simulink model "VFD"  (R2024b)
settings: Solver=VariableStepAuto  StartTime=0.0  StopTime=10/50  RelTol=1e-3
values from neighbouring files (symbols this model uses):
  C = (1-d)/(8*L*(2/31)*freq*freq)    (= 6.25e-05)    [variables.m]
  fnew = 33    [variables.m]
  freq = 50    [variables.m]
  r = 1000    [variables.m]
undefined symbols (not defined in the file or in its folder): Down, Up
libraries: fl_lib x38, nesl_utility x27, ee_lib x12, eePwmGenerator x3, simulink x1
settings Model: Creator=nilab  LastModifiedBy=nilab
settings DebuggingCC: ReadBeforeWriteMsg=DisableAll  WriteAfterWriteMsg=DisableAll  WriteAfterReadMsg=DisableAll  MultiTaskDSMMsg=none
settings ModelReferenceCC: UpdateModelReferenceTargets=IfOutOfDate
settings SFSimCC: SFSimEcho=off

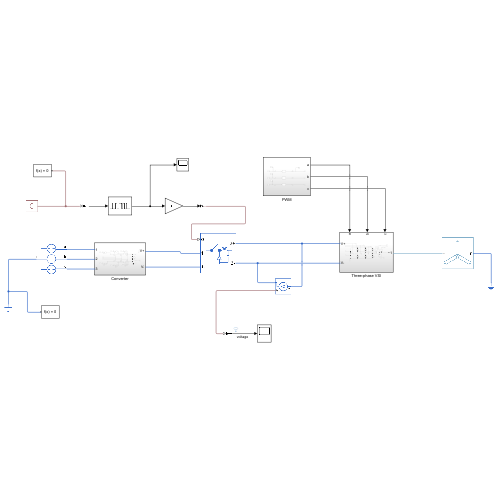
[thumbnail: Simulink's stored preview of the top-level diagram]
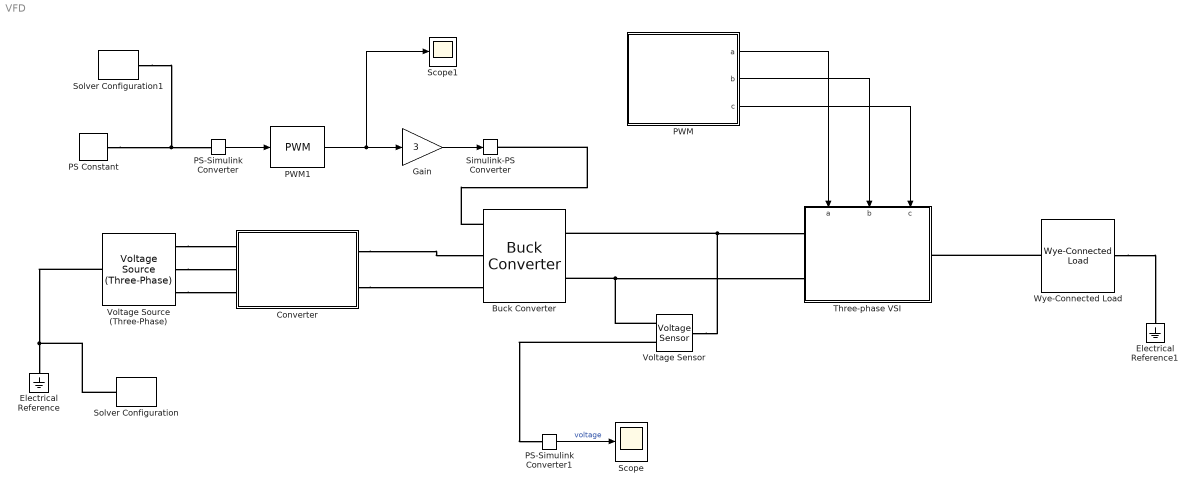
== system VFD ==
  Buck Converter : ee_lib/Semiconductors & Converters/Converters/Buck Converter  port_option=ee.enum.controlport.ps  device_type=ee.enum.converters.switchingdevice.ideal  Vf=0.8 V  Ron=0.001 Ohm  Rds=0.001 Ohm  Goff=1e-5 1/Ohm  Vgt=1 V  Vgt_off=-1 V  Ih=1 A  Vth=2 V  K=0  diode_param=ee.enum.converters.protectiondiode.nodynamics  diode_Vf=0.8 V  diode_Ron=0.001 Ohm  diode_Goff=1e-5 1/Ohm  diode_C=50 nF  diode_iRM=-235 A  diode_iF=300 A  diode_idot=-50 A/us  diode_trr_param=ee.enum.converters.diodetrr.trr_factor  diode_trr_factor=3  diode_trr=15 us  diode_Qrr=1500 s*uA  Lf=L H  Rl=0 Ohm  Cf=C*1e6 uF  Rf=1e-6 Ohm  snubber_type=ee.enum.converters.snubber.exclude  Cs=1e-7 F  Rs=0.1 Ohm  iL_specify=off  iL_priority=High  iL=0 A  iL_nominal_specify=off  iL_nominal_value=1  iL_nominal_unit=A  vc_specify=off  vc_priority=High  vc=0 V  vc_nominal_specify=off  vc_nominal_value=1  vc_nominal_unit=V
      settings: InternalSimscapePortConfiguration="{\"Bottom\":[],\"Left\":[{\"id\":\"G\",\"label\":\"G\",\"type\":\"input\"},{\"id\":\"p1\",\"label\":\"1+\",\"type\":\"foundation.electrical.electrical\"},{\"id\":\"n1\",\"label\":\"1-\",\"type\":\"foundation.electrical.electrical\"}],\"Right\":[{\"id\":\"p2\",\"label\":\"2+\",\"type\":\"foundation.electrical.electrical\"},{\"id\":\"n2\",\"label\":\"2-\",\"type\":\"foundation.electrical.electrical\"}],\"Top\":[]}"
  Converter : Subsystem
  Electrical Reference : fl_lib/Electrical/Electrical Elements/Electrical Reference
  Electrical Reference1 : fl_lib/Electrical/Electrical Elements/Electrical Reference
  Gain : Gain  Gain=3
  PS Constant : fl_lib/Physical Signals/Sources/PS Constant  constant=d
  PS-Simulink Converter : nesl_utility/PS-Simulink Converter  PhysicalDomain=network_engine_domain  SubClassName=ps_output  LeftPortType=input  RightPortType=output  PseudoPeriodic=off  Frequencies=[]  VectorFormat=inherit  Unit=inherit  AffineConversion=off
  PS-Simulink Converter1 : nesl_utility/PS-Simulink Converter  PhysicalDomain=network_engine_domain  SubClassName=ps_output  LeftPortType=input  RightPortType=output  PseudoPeriodic=off  Frequencies=[]  VectorFormat=inherit  Unit=inherit  AffineConversion=off
  PWM : Subsystem
  PWM1 : simulink/Discontinuities/PWM  DisableCoverage=on  Period=1/fnew  InitialDelay=0  DisallowZeroDutyCycle=off  RunAtFixedTimeIntervals=off  SampleTime=0.1
  Scope : Scope
  Scope1 : Scope
  Simulink-PS Converter : nesl_utility/Simulink-PS Converter  PhysicalDomain=network_engine_domain  SubClassName=ps_input  LeftPortType=input  RightPortType=output  PseudoPeriodic=off  Frequencies=[]  NoiseDistribution=none  NoiseParameters=[]  Unit=1  AffineConversion=off  FilteringAndDerivatives=provide  SimscapeFilterOrder=1  InputFilterTimeConstant=0.001  UdotUserProvided=0
  Solver Configuration : nesl_utility/Solver Configuration  PhysicalDomain=network_engine_domain  SubClassName=solver  LeftPortType=input  RightPortType=generic  Tones=[]  Harmonics=[]  SimulateNoise=off  Profile=off  UseLocalSampling=off  EnableSwitchedLinearOptims=on  FrequencyDomain=off  UseCCode=off  RelTol=0.001  AbsTol=0.001  MinStep=1e-09  ToWorkspace=off  RevertToSquareIcSolve=off  NumHomotopyIterations=100  PhasorMode=off  PhasorModeNumHarmonics=1  ConsistencySolver=NEWTON_XTOL_AFTER_FTOL  IndexReductionMethod=DerivativeReplacement  DoDC=off  ResidualTolerance=1e-09  ConsistencyTolSource=GLOBAL  ConsistencyAbsTol=0.001  ConsistencyRelTol=0.001  ConsistencyTolFactor=0.001  UseLocalSolver=off  LocalSolverChoice=NE_BACKWARD_EULER_ADVANCER  ResolveIndetEquations=on  FunctionEvalNumThread=1  LocalSolverSampleTime=0.001  DoFixedCost=off  MaxNonlinIter=3  MaxModeIter=2  ComputeImpulses=off  ImpulseIterations=2  LinearAlgebra=auto  LinearAlgebraNumThread=0  EquationFormulation=NE_TIME_EF  DelaysMemoryBudget=1024  AutomaticFiltering=on  FilteringTimeConstant=0.001  PartitionStorageMethod=AS_NEEDED  PartitionMemoryBudget=1024  PartitionMethod=ROBUST  MultibodyUseLocalSolver=off  MultibodyLocalSolverChoice=ODE1  MultibodyLocalSolverSampleTime=0.001
  Solver Configuration1 : nesl_utility/Solver Configuration  PhysicalDomain=network_engine_domain  SubClassName=solver  LeftPortType=input  RightPortType=generic  Tones=[]  Harmonics=[]  SimulateNoise=off  Profile=off  UseLocalSampling=off  EnableSwitchedLinearOptims=on  FrequencyDomain=off  UseCCode=off  RelTol=0.001  AbsTol=0.001  MinStep=1e-09  ToWorkspace=off  RevertToSquareIcSolve=off  NumHomotopyIterations=100  PhasorMode=off  PhasorModeNumHarmonics=1  ConsistencySolver=NEWTON_XTOL_AFTER_FTOL  IndexReductionMethod=DerivativeReplacement  DoDC=off  ResidualTolerance=1e-09  ConsistencyTolSource=GLOBAL  ConsistencyAbsTol=0.001  ConsistencyRelTol=0.001  ConsistencyTolFactor=0.001  UseLocalSolver=off  LocalSolverChoice=NE_BACKWARD_EULER_ADVANCER  ResolveIndetEquations=on  FunctionEvalNumThread=1  LocalSolverSampleTime=0.001  DoFixedCost=off  MaxNonlinIter=3  MaxModeIter=2  ComputeImpulses=off  ImpulseIterations=2  LinearAlgebra=auto  LinearAlgebraNumThread=0  EquationFormulation=NE_TIME_EF  DelaysMemoryBudget=1024  AutomaticFiltering=on  FilteringTimeConstant=0.001  PartitionStorageMethod=AS_NEEDED  PartitionMemoryBudget=1024  PartitionMethod=ROBUST  MultibodyUseLocalSolver=off  MultibodyLocalSolverChoice=ODE1  MultibodyLocalSolverSampleTime=0.001
  Three-phase VSI : Subsystem
      settings: PortSchema="{\"entries\":[{\"content\":{\"sides\":[{\"content\":{\"connectorIds\":[\"LConn1\",\"LConn2\"]},\"type\":\"ConnectorPlacement.EquallySpacedRectSide\",\"uuid\":\"2b5e637c-93e3-4064-8bf6-4f52f0e07da4\"},{\"content\":{\"connectorIds\":[\"RConn1\"],\"side\":\"RIGHT\"},\"type\":\"ConnectorPlacement.EquallySpacedRectSide\",\"uuid\":\"63a19c73-cdb8-4eaa-8504-93f2b55e949d\"},{\"content\":{\"connectorIds\":[\"In1\",\"In2\",\"In3\"],\"side\":\"TOP\"},\"type\":\"ConnectorPlacement.EquallySpacedRectSide\",\"uuid\":\"d4653da6-a00c-414a-9a01-4f896c6dc2e2\"}]},\"type\":\"ConnectorPlacement.EquallySpacedConnector\",\"uuid\":\"c4601345-6e28-4ab4-9b60-968efd743150\"}],\"packageUris\":[\"http://schema.mathworks.com/mf0/Connector/R2020b\"],\"version\":\"1.0\"}"
  Voltage Source (Three-Phase) : ee_lib/Sources/Voltage Source (Three-Phase)  vline_rms=220/sqrt(3) V  shift=0 deg  freq=50 Hz  impedance_option=1  SShortCircuit=1e6 A*V  XR=15  R=0.01 Ohm  L=3.97e-4 H  harmonic_option=0  harmonic_orders=[5, 7, 11, 13]  harmonic_ratios=[.1, .1, .1, .1]  G_parasitic=0 1/Ohm  I_specify=off  I_priority=None  I=[0, 0, 0] A  I_nominal_specify=off  I_nominal_value=1  I_nominal_unit=A
      settings: InternalSimscapePortConfiguration="{\"Bottom\":[],\"Left\":[{\"id\":\"n\",\"label\":\"n\",\"type\":\"foundation.electrical.electrical\"}],\"Right\":[{\"id\":\"a\",\"label\":\"a\",\"type\":\"foundation.electrical.electrical\"},{\"id\":\"b\",\"label\":\"b\",\"type\":\"foundation.electrical.electrical\"},{\"id\":\"c\",\"label\":\"c\",\"type\":\"foundation.electrical.electrical\"}],\"Top\":[]}"
  Voltage Sensor : fl_lib/Electrical/Electrical Sensors/Voltage Sensor
  Wye-Connected Load : ee_lib/Passive/RLC Assemblies/Wye-Connected Load  port_option=ee.enum.threePhasePort.composite  parameterization=ee.enum.rlc.parameterization.direct  component_structure=ee.enum.rlc.structure.R  component_structure_PQ=ee.enum.rlc.structure.R  R=r Ohm  L=1e-3 H  C=1e-6 F  VRated=24e3 V  FRated=60 Hz  P=1e3 W  Qpos=1e2 A*V  Qneg=-1e2 A*V  R_parasitic=1e-6 Ohm  G_parasitic=1e-6 1/Ohm  R_parasitic_PQ=1e-6 Ohm  G_parasitic_PQ=1e-6 1/Ohm  Vmag0=24e3 V  Vang0=0 deg  Freq0=60 Hz  IL_specify=off  IL_priority=High  IL=[0, 0, 0] A  IL_nominal_specify=off  IL_nominal_value=1  IL_nominal_unit=A  VC_specify=off  VC_priority=High  VC=[0, 0, 0] V  VC_nominal_specify=off  VC_nominal_value=1  VC_nominal_unit=V
  wires:
  PS-Simulink Converter/1 -> PWM1/1
  PWM/1(a) -> Three-phase VSI/1(a)
  PWM/2(b) -> Three-phase VSI/2(b)
  PWM/3(c) -> Three-phase VSI/3(c)
  PS-Simulink Converter1/1 -> Scope/1  "voltage"
  PWM1/1 -> Gain/1, Scope1/1
  Gain/1 -> Simulink-PS Converter/1
  connections:
  Voltage Source (Three-Phase)/RConn2 -- Converter/LConn2
  Voltage Source (Three-Phase)/RConn1 -- Converter/LConn1
  Voltage Source (Three-Phase)/RConn3 -- Converter/LConn3
  Voltage Source (Three-Phase)/LConn1 -- Solver Configuration/RConn1 -- Electrical Reference/LConn1
  Buck Converter/LConn1 -- Simulink-PS Converter/RConn1
  PS Constant/RConn1 -- PS-Simulink Converter/LConn1 -- Solver Configuration1/RConn1
  Voltage Sensor/RConn2 -- Three-phase VSI/LConn2 -- Buck Converter/RConn2
  Voltage Sensor/RConn1 -- PS-Simulink Converter1/LConn1
  Voltage Sensor/LConn1 -- Three-phase VSI/LConn1 -- Buck Converter/RConn1
  Converter/RConn2 -- Buck Converter/LConn3
  Converter/RConn1 -- Buck Converter/LConn2
  Wye-Connected Load/LConn1 -- Three-phase VSI/RConn1
  Wye-Connected Load/RConn1 -- Electrical Reference1/LConn1

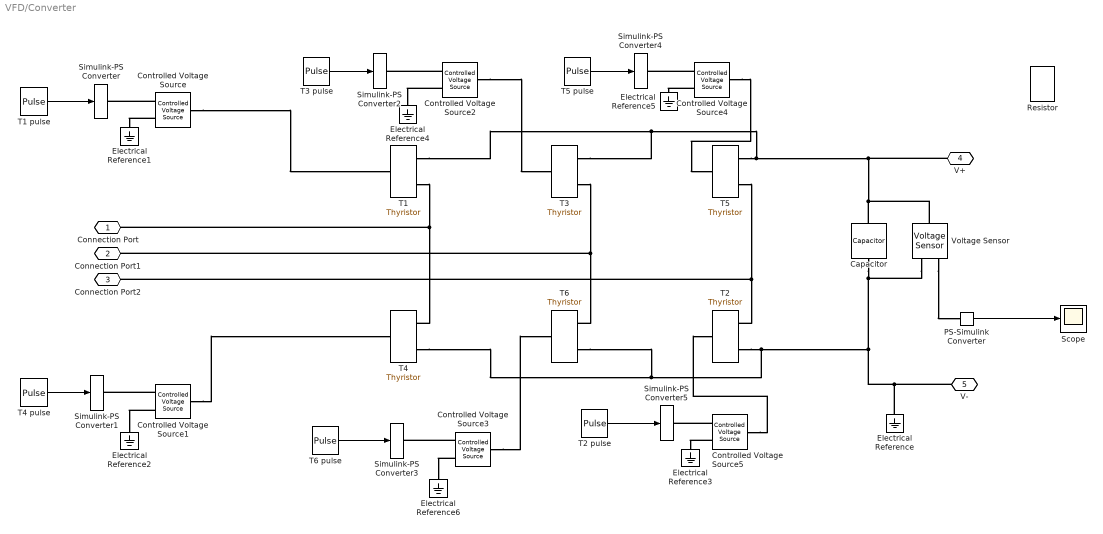
== system VFD/Converter ==
  Capacitor : fl_lib/Electrical/Electrical Elements/Capacitor  c=100 uF  r=1e-6 Ohm  g=0 1/Ohm  i_specify=off  i_priority=None  i=0 A  i_nominal_specify=off  i_nominal_value=1  i_nominal_unit=A  v_specify=off  v_priority=None  v=0 V  v_nominal_specify=off  v_nominal_value=1  v_nominal_unit=V  vc_specify=off  vc_priority=High  vc=0 V  vc_nominal_specify=off  vc_nominal_value=1  vc_nominal_unit=V
  Controlled Voltage Source{,1..5} (6 alike) : fl_lib/Electrical/Electrical Sources/Controlled Voltage Source
  Electrical Reference{,1..6} (7 alike) : fl_lib/Electrical/Electrical Elements/Electrical Reference
  PS-Simulink Converter : nesl_utility/PS-Simulink Converter  PhysicalDomain=network_engine_domain  SubClassName=ps_output  LeftPortType=input  RightPortType=output  PseudoPeriodic=off  Frequencies=[]  VectorFormat=inherit  Unit=inherit  AffineConversion=off
  Resistor : fl_lib/Electrical/Electrical Elements/Resistor  R=1 Ohm  i_specify=off  i_priority=None  i=0 A  i_nominal_specify=off  i_nominal_value=1  i_nominal_unit=A  v_specify=off  v_priority=None  v=0 V  v_nominal_specify=off  v_nominal_value=1  v_nominal_unit=V
  Scope : Scope
  Simulink-PS Converter{,1..5} (6 alike) : nesl_utility/Simulink-PS Converter  PhysicalDomain=network_engine_domain  SubClassName=ps_input  LeftPortType=input  RightPortType=output  PseudoPeriodic=off  Frequencies=[]  NoiseDistribution=none  NoiseParameters=[]  Unit=1  AffineConversion=off  FilteringAndDerivatives=zero  SimscapeFilterOrder=1  InputFilterTimeConstant=0.001  UdotUserProvided=1
  T{1..6} (6 alike) : ee_lib/Semiconductors & Converters/Thyristor  model_type=ee.enum.semiconductors.thyristorModelType.equations  v_on=1.2 V  i_on=1 A  VT_vec=[.75, 1, 1.25, 1.5, 1.75, 2, 2.25] V  IT_vec=[.015, .22, .75, 1.4, 2, 2.75, 3.45] A  IDRM=0.01 mA  VDRM=400 V  i_H=1 mA  Tmeas=25 degC  i_GT=3 uA  v_GT=0.6 V  V_D=12 V  R=120 Ohm  dVdt=150 V/us  R_GK=1000 Ohm  TF_NPN_parameterization=1  T_d=2 us  i_d=10 mA  TF_NPN=0.3 us  TF_PNP_parameterization=1  TF_PNP=0.3 us  t_on_delay=0 s  t_on_curr=1 mA  t_on_rise=0 s  Rs=87 kOhm  Rgate=10 Ohm  Gain=10  ig_specify=off  ig_priority=None  ig=0 A  ig_nominal_specify=off  ig_nominal_value=1  ig_nominal_unit=A  ia_specify=off  ia_priority=None  ia=0 A  ia_nominal_specify=off  ia_nominal_value=1  ia_nominal_unit=A  vgk_specify=off  vgk_priority=None  vgk=0 V  vgk_nominal_specify=off  vgk_nominal_value=1  vgk_nominal_unit=V  vak_specify=off  vak_priority=None  vak=0 V  vak_nominal_specify=off  vak_nominal_value=1  vak_nominal_unit=V  Q_npn_bc_specify=off  Q_npn_bc_priority=High  Q_npn_bc=0 C  Q_npn_bc_nominal_specify=off  Q_npn_bc_nominal_value=1  Q_npn_bc_nominal_unit=uC  Q_npn_be_specify=off  Q_npn_be_priority=High  Q_npn_be=0 C  Q_npn_be_nominal_specify=off  Q_npn_be_nominal_value=1  Q_npn_be_nominal_unit=uC  Q_pnp_be_specify=off  Q_pnp_be_priority=High  Q_pnp_be=0 C  Q_pnp_be_nominal_specify=off  Q_pnp_be_nominal_value=1  Q_pnp_be_nominal_unit=uC  thermal_network_parameterization=ee.enum.thermalNetworkTopology.junctionCase  Rth=[0, 10] K/W  Rth_Cauer=[1, 3, 10] K/W  Rth_Foster=[4, 6] K/W  thermal_mass_parameterization=ee.enum.thermalNetwork.timeconstant  thermal_mass=[0, 1] J/K  thermal_mass_Cauer=[.1, .3, 1] J/K  thermal_mass_Foster=[1.5, 3] J/K  thermal_time_constant=[0, 10] s  thermal_time_constant_Cauer=[1, 3, 10] s  thermal_time_constant_Foster=[6, 18] s  thermal_mass_initial_temperatures=[25, 25] degC  thermal_mass_initial_temperatures_Cauer=[25, 25, 25] degC  Tvec_initial_Foster=[25, 25, 25, 25] degC
      settings: InternalSimscapePortConfiguration="{\"Bottom\":[],\"Left\":[{\"id\":\"G\",\"label\":\"\",\"type\":\"foundation.electrical.electrical\"}],\"Right\":[{\"id\":\"A\",\"label\":\"\",\"type\":\"foundation.electrical.electrical\"},{\"id\":\"K\",\"label\":\"\",\"type\":\"foundation.electrical.electrical\"}],\"Top\":[]}"
  T1 pulse : DiscretePulseGenerator  PulseType=Time based  Amplitude=2  Period=1/freq  PulseWidth=5  PhaseDelay=1/(12*freq)
  T2 pulse : DiscretePulseGenerator  PulseType=Time based  Amplitude=2  Period=1/freq  PulseWidth=5  PhaseDelay=1/(4*freq)
  T3 pulse : DiscretePulseGenerator  PulseType=Time based  Amplitude=2  Period=1/freq  PulseWidth=5  PhaseDelay=5/(12*freq)
  T4 pulse : DiscretePulseGenerator  PulseType=Time based  Amplitude=2  Period=1/freq  PulseWidth=5  PhaseDelay=7/(12*freq)
  T5 pulse : DiscretePulseGenerator  PulseType=Time based  Amplitude=2  Period=1/freq  PulseWidth=5  PhaseDelay=3/(4*freq)
  T6 pulse : DiscretePulseGenerator  PulseType=Time based  Amplitude=2  Period=1/freq  PulseWidth=5  PhaseDelay=11/(12*freq)
  Voltage Sensor : fl_lib/Electrical/Electrical Sensors/Voltage Sensor
  Connection Port : PMIOPort  Side=Left
  Connection Port1 : PMIOPort  Port=2  Side=Left
  Connection Port2 : PMIOPort  Port=3  Side=Left
  V+ : PMIOPort  Port=4  Side=Right
  V- : PMIOPort  Port=5  Side=Right
  wires:
  T1 pulse/1 -> Simulink-PS Converter/1
  T6 pulse/1 -> Simulink-PS Converter3/1
  T5 pulse/1 -> Simulink-PS Converter4/1
  T2 pulse/1 -> Simulink-PS Converter5/1
  T3 pulse/1 -> Simulink-PS Converter2/1
  PS-Simulink Converter/1 -> Scope/1
  T4 pulse/1 -> Simulink-PS Converter1/1
  connections:
  T5/RConn1 -- Connection Port2/RConn1 -- T2/RConn2
  T6/RConn2 -- Connection Port1/RConn1 -- T3/RConn1
  T1/RConn1 -- T4/RConn2 -- Connection Port/RConn1
  Controlled Voltage Source5/LConn1 -- T2/LConn1
  Controlled Voltage Source3/RConn2 -- Electrical Reference6/LConn1
  Voltage Sensor/RConn1 -- PS-Simulink Converter/LConn1
  Controlled Voltage Source1/RConn1 -- Simulink-PS Converter1/RConn1
  Controlled Voltage Source5/RConn1 -- Simulink-PS Converter5/RConn1
  Controlled Voltage Source4/RConn2 -- Electrical Reference5/LConn1
  Controlled Voltage Source3/RConn1 -- Simulink-PS Converter3/RConn1
  Controlled Voltage Source4/LConn1 -- T5/LConn1
  Controlled Voltage Source3/LConn1 -- T6/LConn1
  Controlled Voltage Source1/LConn1 -- T4/LConn1
  Controlled Voltage Source5/RConn2 -- Electrical Reference3/LConn1
  Controlled Voltage Source2/RConn1 -- Simulink-PS Converter2/RConn1
  Controlled Voltage Source/RConn2 -- Electrical Reference1/LConn1
  Controlled Voltage Source1/RConn2 -- Electrical Reference2/LConn1
  Controlled Voltage Source2/LConn1 -- T3/LConn1
  Controlled Voltage Source4/RConn1 -- Simulink-PS Converter4/RConn1
  Controlled Voltage Source2/RConn2 -- Electrical Reference4/LConn1
  Controlled Voltage Source/RConn1 -- Simulink-PS Converter/RConn1
  Controlled Voltage Source/LConn1 -- T1/LConn1
  T6/RConn1 -- T4/RConn1 -- Electrical Reference/LConn1 -- V-/RConn1 -- Capacitor/RConn1 -- Voltage Sensor/RConn2 -- T2/RConn1
  T3/RConn2 -- T1/RConn2 -- V+/RConn1 -- Capacitor/LConn1 -- Voltage Sensor/LConn1 -- T5/RConn2

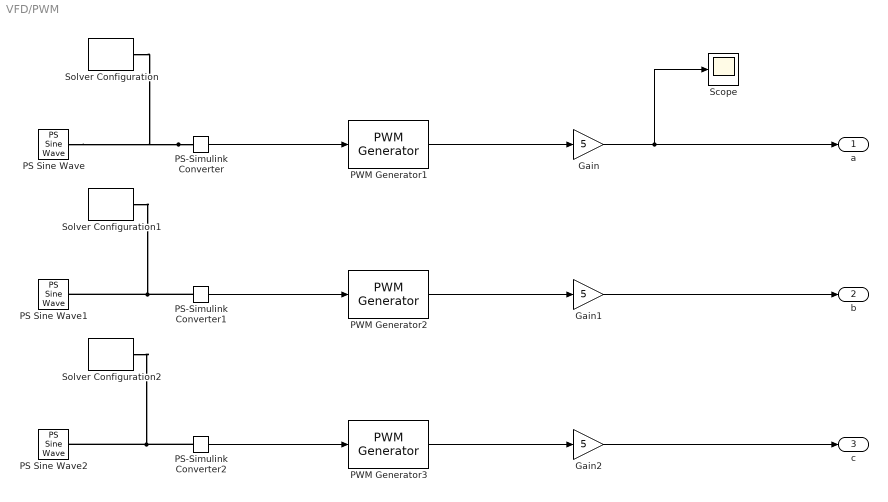
== system VFD/PWM ==
  Gain : Gain  Gain=5
  Gain1 : Gain  Gain=5
  Gain2 : Gain  Gain=5
  PS Sine Wave : fl_lib/Physical Signals/Sources/PS Sine Wave  amplitude=1  bias=0  frequency_spec=foundation.enum.frequencySpec.frequencySI  frequency_SI=fnew Hz  frequency_angular=1 rad/s  phase=0 rad
      settings: InternalSimscapePortConfiguration="{\"Bottom\":[],\"Left\":[],\"Right\":[{\"id\":\"O\",\"label\":\"\",\"type\":\"output\"}],\"Top\":[]}"
  PS Sine Wave1 : fl_lib/Physical Signals/Sources/PS Sine Wave  amplitude=1  bias=0  frequency_spec=foundation.enum.frequencySpec.frequencySI  frequency_SI=fnew Hz  frequency_angular=1 rad/s  phase=-120 deg
      settings: InternalSimscapePortConfiguration="{\"Bottom\":[],\"Left\":[],\"Right\":[{\"id\":\"O\",\"label\":\"\",\"type\":\"output\"}],\"Top\":[]}"
  PS Sine Wave2 : fl_lib/Physical Signals/Sources/PS Sine Wave  amplitude=1  bias=0  frequency_spec=foundation.enum.frequencySpec.frequencySI  frequency_SI=fnew Hz  frequency_angular=1 rad/s  phase=120 deg
      settings: InternalSimscapePortConfiguration="{\"Bottom\":[],\"Left\":[],\"Right\":[{\"id\":\"O\",\"label\":\"\",\"type\":\"output\"}],\"Top\":[]}"
  PS-Simulink Converter : nesl_utility/PS-Simulink Converter  PhysicalDomain=network_engine_domain  SubClassName=ps_output  LeftPortType=input  RightPortType=output  PseudoPeriodic=off  Frequencies=[]  VectorFormat=inherit  Unit=inherit  AffineConversion=off
  PS-Simulink Converter1 : nesl_utility/PS-Simulink Converter  PhysicalDomain=network_engine_domain  SubClassName=ps_output  LeftPortType=input  RightPortType=output  PseudoPeriodic=off  Frequencies=[]  VectorFormat=inherit  Unit=inherit  AffineConversion=off
  PS-Simulink Converter2 : nesl_utility/PS-Simulink Converter  PhysicalDomain=network_engine_domain  SubClassName=ps_output  LeftPortType=input  RightPortType=output  PseudoPeriodic=off  Frequencies=[]  VectorFormat=inherit  Unit=inherit  AffineConversion=off
  PWM Generator1 : eePwmGenerator/PWM Generator  CarrCount=Up-Down  Tper=0.0005  Tdelay=0  Ts=0
  PWM Generator2 : eePwmGenerator/PWM Generator  CarrCount=Up-Down  Tper=0.0005  Tdelay=0  Ts=0
  PWM Generator3 : eePwmGenerator/PWM Generator  CarrCount=Up-Down  Tper=0.0005  Tdelay=0  Ts=0
  Scope : Scope
  Solver Configuration : nesl_utility/Solver Configuration  PhysicalDomain=network_engine_domain  SubClassName=solver  LeftPortType=input  RightPortType=generic  Tones=[]  Harmonics=[]  SimulateNoise=off  Profile=off  UseLocalSampling=off  EnableSwitchedLinearOptims=on  FrequencyDomain=off  UseCCode=off  RelTol=0.001  AbsTol=0.001  MinStep=1e-09  ToWorkspace=off  RevertToSquareIcSolve=off  NumHomotopyIterations=100  PhasorMode=off  PhasorModeNumHarmonics=1  ConsistencySolver=NEWTON_XTOL_AFTER_FTOL  IndexReductionMethod=DerivativeReplacement  DoDC=off  ResidualTolerance=1e-09  ConsistencyTolSource=GLOBAL  ConsistencyAbsTol=0.001  ConsistencyRelTol=0.001  ConsistencyTolFactor=0.001  UseLocalSolver=off  LocalSolverChoice=NE_BACKWARD_EULER_ADVANCER  ResolveIndetEquations=on  FunctionEvalNumThread=1  LocalSolverSampleTime=0.001  DoFixedCost=off  MaxNonlinIter=3  MaxModeIter=2  ComputeImpulses=off  ImpulseIterations=2  LinearAlgebra=auto  LinearAlgebraNumThread=0  EquationFormulation=NE_TIME_EF  DelaysMemoryBudget=1024  AutomaticFiltering=on  FilteringTimeConstant=0.001  PartitionStorageMethod=AS_NEEDED  PartitionMemoryBudget=1024  PartitionMethod=ROBUST  MultibodyUseLocalSolver=off  MultibodyLocalSolverChoice=ODE1  MultibodyLocalSolverSampleTime=0.001
  Solver Configuration1 : nesl_utility/Solver Configuration  PhysicalDomain=network_engine_domain  SubClassName=solver  LeftPortType=input  RightPortType=generic  Tones=[]  Harmonics=[]  SimulateNoise=off  Profile=off  UseLocalSampling=off  EnableSwitchedLinearOptims=on  FrequencyDomain=off  UseCCode=off  RelTol=0.001  AbsTol=0.001  MinStep=1e-09  ToWorkspace=off  RevertToSquareIcSolve=off  NumHomotopyIterations=100  PhasorMode=off  PhasorModeNumHarmonics=1  ConsistencySolver=NEWTON_XTOL_AFTER_FTOL  IndexReductionMethod=DerivativeReplacement  DoDC=off  ResidualTolerance=1e-09  ConsistencyTolSource=GLOBAL  ConsistencyAbsTol=0.001  ConsistencyRelTol=0.001  ConsistencyTolFactor=0.001  UseLocalSolver=off  LocalSolverChoice=NE_BACKWARD_EULER_ADVANCER  ResolveIndetEquations=on  FunctionEvalNumThread=1  LocalSolverSampleTime=0.001  DoFixedCost=off  MaxNonlinIter=3  MaxModeIter=2  ComputeImpulses=off  ImpulseIterations=2  LinearAlgebra=auto  LinearAlgebraNumThread=0  EquationFormulation=NE_TIME_EF  DelaysMemoryBudget=1024  AutomaticFiltering=on  FilteringTimeConstant=0.001  PartitionStorageMethod=AS_NEEDED  PartitionMemoryBudget=1024  PartitionMethod=ROBUST  MultibodyUseLocalSolver=off  MultibodyLocalSolverChoice=ODE1  MultibodyLocalSolverSampleTime=0.001
  Solver Configuration2 : nesl_utility/Solver Configuration  PhysicalDomain=network_engine_domain  SubClassName=solver  LeftPortType=input  RightPortType=generic  Tones=[]  Harmonics=[]  SimulateNoise=off  Profile=off  UseLocalSampling=off  EnableSwitchedLinearOptims=on  FrequencyDomain=off  UseCCode=off  RelTol=0.001  AbsTol=0.001  MinStep=1e-09  ToWorkspace=off  RevertToSquareIcSolve=off  NumHomotopyIterations=100  PhasorMode=off  PhasorModeNumHarmonics=1  ConsistencySolver=NEWTON_XTOL_AFTER_FTOL  IndexReductionMethod=DerivativeReplacement  DoDC=off  ResidualTolerance=1e-09  ConsistencyTolSource=GLOBAL  ConsistencyAbsTol=0.001  ConsistencyRelTol=0.001  ConsistencyTolFactor=0.001  UseLocalSolver=off  LocalSolverChoice=NE_BACKWARD_EULER_ADVANCER  ResolveIndetEquations=on  FunctionEvalNumThread=1  LocalSolverSampleTime=0.001  DoFixedCost=off  MaxNonlinIter=3  MaxModeIter=2  ComputeImpulses=off  ImpulseIterations=2  LinearAlgebra=auto  LinearAlgebraNumThread=0  EquationFormulation=NE_TIME_EF  DelaysMemoryBudget=1024  AutomaticFiltering=on  FilteringTimeConstant=0.001  PartitionStorageMethod=AS_NEEDED  PartitionMemoryBudget=1024  PartitionMethod=ROBUST  MultibodyUseLocalSolver=off  MultibodyLocalSolverChoice=ODE1  MultibodyLocalSolverSampleTime=0.001
  a : Outport
  b : Outport  Port=2
  c : Outport  Port=3
  wires:
  PS-Simulink Converter/1 -> PWM Generator1/1
  PS-Simulink Converter1/1 -> PWM Generator2/1
  PS-Simulink Converter2/1 -> PWM Generator3/1
  PWM Generator1/1 -> Gain/1
  PWM Generator2/1 -> Gain1/1
  PWM Generator3/1 -> Gain2/1
  Gain/1 -> a/1, Scope/1
  Gain1/1 -> b/1
  Gain2/1 -> c/1
  connections:
  PS-Simulink Converter1/LConn1 -- PS Sine Wave1/RConn1 -- Solver Configuration1/RConn1
  PS-Simulink Converter2/LConn1 -- Solver Configuration2/RConn1 -- PS Sine Wave2/RConn1
  PS-Simulink Converter/LConn1 -- PS Sine Wave/RConn1 -- Solver Configuration/RConn1

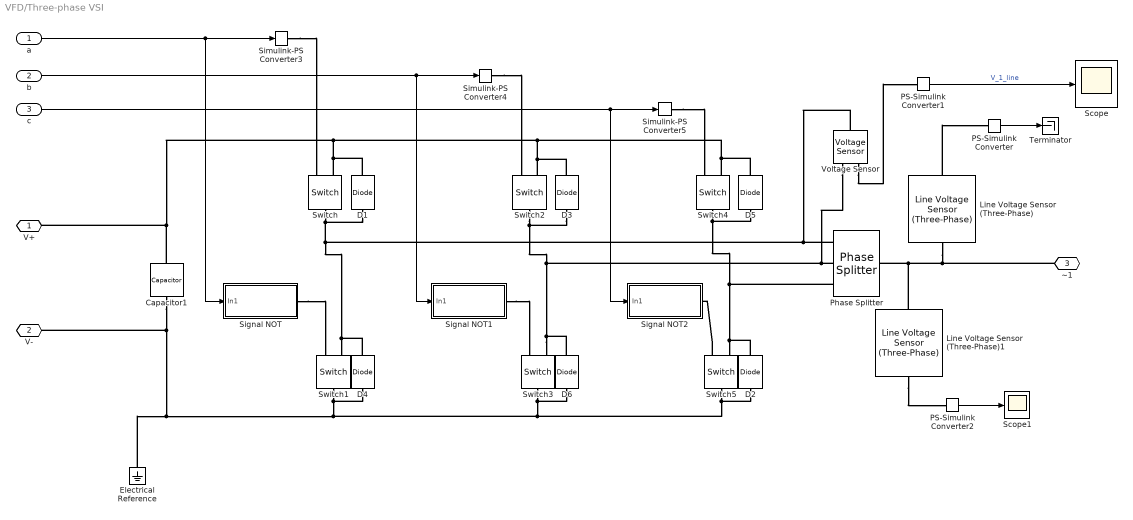
== system VFD/Three-phase VSI ==
  a : Inport
  b : Inport  Port=2
  c : Inport  Port=3
  Capacitor1 : fl_lib/Electrical/Electrical Elements/Capacitor  c=50 pF  r=1e-3 mOhm  g=0 1/Ohm  i_specify=off  i_priority=None  i=0 A  i_nominal_specify=off  i_nominal_value=1  i_nominal_unit=A  v_specify=off  v_priority=None  v=0 V  v_nominal_specify=off  v_nominal_value=1  v_nominal_unit=V  vc_specify=off  vc_priority=High  vc=0 V  vc_nominal_specify=off  vc_nominal_value=1  vc_nominal_unit=V
  D{1..6} (6 alike) : fl_lib/Electrical/Electrical Elements/Diode  Vf=0.6 V  Ron=0.3 Ohm  Goff=1e-8 1/Ohm  i_specify=off  i_priority=None  i=0 A  i_nominal_specify=off  i_nominal_value=1  i_nominal_unit=A  v_specify=off  v_priority=None  v=0 V  v_nominal_specify=off  v_nominal_value=1  v_nominal_unit=V
  Electrical Reference : fl_lib/Electrical/Electrical Elements/Electrical Reference
  Line Voltage Sensor (Three-Phase) : ee_lib/Sensors & Transducers/Line Voltage Sensor (Three-Phase)
  Line Voltage Sensor (Three-Phase)1 : ee_lib/Sensors & Transducers/Line Voltage Sensor (Three-Phase)
  PS-Simulink Converter : nesl_utility/PS-Simulink Converter  PhysicalDomain=network_engine_domain  SubClassName=ps_output  LeftPortType=input  RightPortType=output  PseudoPeriodic=off  Frequencies=[]  VectorFormat=inherit  Unit=inherit  AffineConversion=off
  PS-Simulink Converter1 : nesl_utility/PS-Simulink Converter  PhysicalDomain=network_engine_domain  SubClassName=ps_output  LeftPortType=input  RightPortType=output  PseudoPeriodic=off  Frequencies=[]  VectorFormat=inherit  Unit=inherit  AffineConversion=off
  PS-Simulink Converter2 : nesl_utility/PS-Simulink Converter  PhysicalDomain=network_engine_domain  SubClassName=ps_output  LeftPortType=input  RightPortType=output  PseudoPeriodic=off  Frequencies=[]  VectorFormat=inherit  Unit=inherit  AffineConversion=off
  Phase Splitter : ee_lib/Connectors & References/Phase Splitter
  Scope : Scope
  Scope1 : Scope
  Signal NOT : Subsystem
  Signal NOT1 : Subsystem
  Signal NOT2 : Subsystem
  Simulink-PS Converter3 : nesl_utility/Simulink-PS Converter  PhysicalDomain=network_engine_domain  SubClassName=ps_input  LeftPortType=input  RightPortType=output  PseudoPeriodic=off  Frequencies=[]  NoiseDistribution=none  NoiseParameters=[]  Unit=1  AffineConversion=off  FilteringAndDerivatives=provide  SimscapeFilterOrder=1  InputFilterTimeConstant=0.001  UdotUserProvided=0
  Simulink-PS Converter4 : nesl_utility/Simulink-PS Converter  PhysicalDomain=network_engine_domain  SubClassName=ps_input  LeftPortType=input  RightPortType=output  PseudoPeriodic=off  Frequencies=[]  NoiseDistribution=none  NoiseParameters=[]  Unit=1  AffineConversion=off  FilteringAndDerivatives=provide  SimscapeFilterOrder=1  InputFilterTimeConstant=0.001  UdotUserProvided=0
  Simulink-PS Converter5 : nesl_utility/Simulink-PS Converter  PhysicalDomain=network_engine_domain  SubClassName=ps_input  LeftPortType=input  RightPortType=output  PseudoPeriodic=off  Frequencies=[]  NoiseDistribution=none  NoiseParameters=[]  Unit=1  AffineConversion=off  FilteringAndDerivatives=provide  SimscapeFilterOrder=1  InputFilterTimeConstant=0.001  UdotUserProvided=0
  Switch{,1..5} (6 alike) : fl_lib/Electrical/Electrical Elements/Switch  R_closed=0.01 Ohm  G_open=1e-8 1/Ohm  Threshold=1.7  i_specify=off  i_priority=None  i=0 A  i_nominal_specify=off  i_nominal_value=1  i_nominal_unit=A  v_specify=off  v_priority=None  v=0 V  v_nominal_specify=off  v_nominal_value=1  v_nominal_unit=V
  Terminator : Terminator
  Voltage Sensor : fl_lib/Electrical/Electrical Sensors/Voltage Sensor
  V+ : PMIOPort  Side=Left
  V- : PMIOPort  Port=2  Side=Left
  ~1 : PMIOPort  Port=3  Side=Right
  wires:
  PS-Simulink Converter1/1 -> Scope/1  "V_1_line"
  c/1 -> Simulink-PS Converter5/1, Signal NOT2/1(In1)
  a/1 -> Signal NOT/1(In1), Simulink-PS Converter3/1
  b/1 -> Signal NOT1/1(In1), Simulink-PS Converter4/1
  PS-Simulink Converter/1 -> Terminator/1
  PS-Simulink Converter2/1 -> Scope1/1
  connections:
  Line Voltage Sensor (Three-Phase)/LConn1 -- Phase Splitter/LConn1 -- Line Voltage Sensor (Three-Phase)1/LConn1 -- ~1/RConn1
  Capacitor1/LConn1 -- D1/RConn1 -- Switch/RConn2 -- D5/RConn1 -- Switch4/RConn2 -- D3/RConn1 -- Switch2/RConn2 -- V+/RConn1
  Capacitor1/RConn1 -- Electrical Reference/LConn1 -- D2/LConn1 -- Switch5/LConn1 -- D6/LConn1 -- Switch3/LConn1 -- D4/LConn1 -- Switch1/LConn1 -- V-/RConn1
  D1/LConn1 -- Switch/LConn1 -- Phase Splitter/RConn1 -- Voltage Sensor/LConn1 -- D4/RConn1 -- Switch1/RConn2
  Switch5/RConn2 -- Phase Splitter/RConn3 -- D5/LConn1 -- Switch4/LConn1 -- D2/RConn1
  Switch3/RConn2 -- D6/RConn1 -- Voltage Sensor/RConn2 -- Phase Splitter/RConn2 -- D3/LConn1 -- Switch2/LConn1
  Simulink-PS Converter4/RConn1 -- Switch2/RConn1
  Simulink-PS Converter5/RConn1 -- Switch4/RConn1
  Line Voltage Sensor (Three-Phase)/RConn1 -- PS-Simulink Converter/LConn1
  Signal NOT/RConn1 -- Switch1/RConn1
  Simulink-PS Converter3/RConn1 -- Switch/RConn1
  Signal NOT1/RConn1 -- Switch3/RConn1
  Voltage Sensor/RConn1 -- PS-Simulink Converter1/LConn1
  Switch5/RConn1 -- Signal NOT2/RConn1
  Line Voltage Sensor (Three-Phase)1/RConn1 -- PS-Simulink Converter2/LConn1

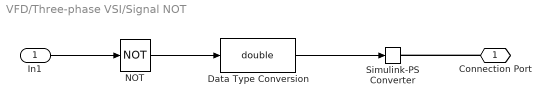
== system VFD/Three-phase VSI/Signal NOT ==
  In1 : Inport
  Data Type Conversion : DataTypeConversion  OutDataTypeStr=double  SaturateOnIntegerOverflow=off  RndMeth=Floor
  NOT : Logic  Operator=NOT  IconShape=distinctive  AllPortsSameDT=off  OutDataTypeStr=boolean
  Simulink-PS Converter : nesl_utility/Simulink-PS Converter  PhysicalDomain=network_engine_domain  SubClassName=ps_input  LeftPortType=input  RightPortType=output  PseudoPeriodic=off  Frequencies=[]  NoiseDistribution=none  NoiseParameters=[]  Unit=1  AffineConversion=off  FilteringAndDerivatives=provide  SimscapeFilterOrder=1  InputFilterTimeConstant=0.001  UdotUserProvided=0
  Connection Port : PMIOPort  Side=Right
  wires:
  In1/1 -> NOT/1
  NOT/1 -> Data Type Conversion/1
  Data Type Conversion/1 -> Simulink-PS Converter/1
  connections:
  Connection Port/RConn1 -- Simulink-PS Converter/RConn1

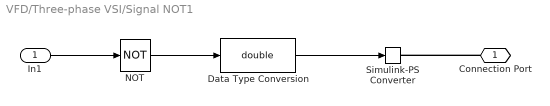
== system VFD/Three-phase VSI/Signal NOT1 ==
  In1 : Inport
  Data Type Conversion : DataTypeConversion  OutDataTypeStr=double  SaturateOnIntegerOverflow=off  RndMeth=Floor
  NOT : Logic  Operator=NOT  IconShape=distinctive  AllPortsSameDT=off  OutDataTypeStr=boolean
  Simulink-PS Converter : nesl_utility/Simulink-PS Converter  PhysicalDomain=network_engine_domain  SubClassName=ps_input  LeftPortType=input  RightPortType=output  PseudoPeriodic=off  Frequencies=[]  NoiseDistribution=none  NoiseParameters=[]  Unit=1  AffineConversion=off  FilteringAndDerivatives=provide  SimscapeFilterOrder=1  InputFilterTimeConstant=0.001  UdotUserProvided=0
  Connection Port : PMIOPort  Side=Right
  wires:
  In1/1 -> NOT/1
  NOT/1 -> Data Type Conversion/1
  Data Type Conversion/1 -> Simulink-PS Converter/1
  connections:
  Connection Port/RConn1 -- Simulink-PS Converter/RConn1

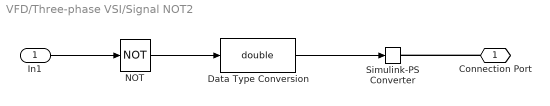
== system VFD/Three-phase VSI/Signal NOT2 ==
  In1 : Inport
  Data Type Conversion : DataTypeConversion  OutDataTypeStr=double  SaturateOnIntegerOverflow=off  RndMeth=Floor
  NOT : Logic  Operator=NOT  IconShape=distinctive  AllPortsSameDT=off  OutDataTypeStr=boolean
  Simulink-PS Converter : nesl_utility/Simulink-PS Converter  PhysicalDomain=network_engine_domain  SubClassName=ps_input  LeftPortType=input  RightPortType=output  PseudoPeriodic=off  Frequencies=[]  NoiseDistribution=none  NoiseParameters=[]  Unit=1  AffineConversion=off  FilteringAndDerivatives=provide  SimscapeFilterOrder=1  InputFilterTimeConstant=0.001  UdotUserProvided=0
  Connection Port : PMIOPort  Side=Right
  wires:
  In1/1 -> NOT/1
  NOT/1 -> Data Type Conversion/1
  Data Type Conversion/1 -> Simulink-PS Converter/1
  connections:
  Connection Port/RConn1 -- Simulink-PS Converter/RConn1
